simulink model "VR_acquisition_serial"  (Simulink 8.4)
settings: Solver=ode45  StartTime=0.0  StopTime=inf  RelTol=1e-3
libraries: vrlib x8, aerolibtransform2 x4, aerolibconvert2 x3
settings Model: Creator=AMANALLAH  LastModifiedBy=AMANALLAH
settings DataIOCC: SignalLoggingSaveFormat=Dataset
settings OptimizationCC: ExpressionDepthLimit=128
settings DebuggingCC: UnderspecifiedInitializationDetection=Simplified  MergeDetectMultiDrivingBlocksExec=error  FcnCallInpInsideContextMsg=EnableAllAsError  StateNameClashWarn=none
settings GRTTargetCC: CombineOutputUpdateFcns=on  GRTInterface=off

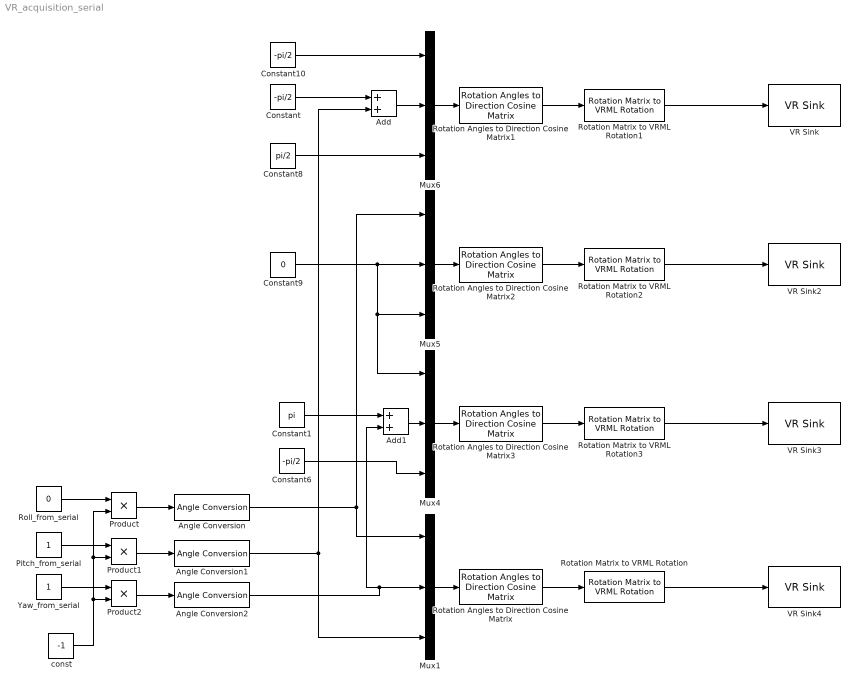
== system VR_acquisition_serial ==
  Add : Sum
  Add1 : Sum
  Angle Conversion : aerolibconvert2/Angle Conversion  IU=deg  OU=rad
  Angle Conversion1 : aerolibconvert2/Angle Conversion  IU=deg  OU=rad
  Angle Conversion2 : aerolibconvert2/Angle Conversion  IU=deg  OU=rad
  Constant : Constant  Value=-pi/2
  Constant1 : Constant  Value=pi
  Constant10 : Constant  Value=-pi/2
  Constant6 : Constant  Value=-pi/2
  Constant8 : Constant  Value=pi/2
  Constant9 : Constant  Value=0
  Mux{1,4..6} (4 alike) : Mux  Inputs=3
  Pitch_from_serial : Constant
  Product : Product
  Product1 : Product
  Product2 : Product
  Roll_from_serial : Constant  Value=0
  Rotation Angles to Direction Cosine Matrix{,1..3} (4 alike) : aerolibtransform2/Rotation Angles to Direction Cosine Matrix  rotationOrder=ZYX
  Rotation Matrix to VRML Rotation{,1..3} (4 alike) : vrlib/Utilities/Rotation Matrix to VRML Rotation  maxzero=1e-12
  VR Sink : vrlib/VR Sink  InstantiateOnLoad=on  SampleTime=0.1  ViewEnable=on  RemoteChange=off  RemoteView=off  FieldsWritten=Airplane.rotation.4.1.1.double  WorldFileName=spitfire_3d_pitch.WRL  AutoView=off  VideoDimensions=[]  AllowVariableSize=off
  VR Sink2 : vrlib/VR Sink  InstantiateOnLoad=on  SampleTime=0.1  ViewEnable=on  RemoteChange=off  RemoteView=off  FieldsWritten=Airplane.rotation.4.1.1.double  WorldFileName=spitfire_3d_roll.WRL  AutoView=off  VideoDimensions=[]  AllowVariableSize=off
  VR Sink3 : vrlib/VR Sink  InstantiateOnLoad=on  SampleTime=0.1  ViewEnable=on  RemoteChange=off  RemoteView=off  FieldsWritten=Airplane.rotation.4.1.1.double  WorldFileName=spitfire_3d_yaw.WRL  AutoView=off  VideoDimensions=[]  AllowVariableSize=off
  VR Sink4 : vrlib/VR Sink  InstantiateOnLoad=on  SampleTime=0.1  ViewEnable=on  RemoteChange=off  RemoteView=off  FieldsWritten=Airplane.rotation.4.1.1.double  WorldFileName=spitfire_3d.WRL  AutoView=off  VideoDimensions=[]  AllowVariableSize=off  FigureProperties="{'Position', 'Name', 'Viewpoint', 'CameraBound', 'CameraDirection', 'CameraPosition', 'CameraUpVector', 'ZoomFactor', 'Antialiasing', 'Headlight', 'Lighting', 'NavPanel', 'Sound', 'StatusBar', 'Stereo3D', 'Stereo3DCameraOffset', 'Stereo3DHIT', 'ToolBar', 'Textures', 'Transparency', 'Triad', 'Wireframe', 'NavZones', 'NavMode', 'NavSpeed', 'CaptureFileFormat', 'CaptureFileName', 'Record2DCompressMethod', 'Record2DCompressQuality', 'Record2D', 'Record2DFileName', 'Record2DFPS'; [4.9900000000000000e+02   1.5700000000000000e+02   5.7600000000000000e+02   3.8000000000000000e+02], '', '_untitled_1', 'on', [0.0000000000000000e+00   0.0000000000000000e+00  -1.0000000000000000e+00], [0.0000000000000000e+00   0.0000000000000000e+00   0.0000000000000000e+00], [0.0000000000000000e+00   1.0000000000000000e+00   0.0000000000000000e+00], [1.0000000000000000e+00], 'on', 'on', 'on', 'halfbar', 'on', 'on', 'off', [1.0000000149011612e-01], [0.0000000000000000e+00], 'on', 'on', 'on', 'none', 'off', 'off', 'fly', 'normal', 'tif', '%f_anim_%n.tif', 'auto', [7.5000000000000000e+01], 'off', '%f_anim_%n.avi', 'auto'}"
  Yaw_from_serial : Constant
  const : Constant  Value=-1
  wires:
  Rotation Matrix to VRML Rotation/1 -> VR Sink4/1
  Rotation Angles to Direction Cosine Matrix/1 -> Rotation Matrix to VRML Rotation/1
  Mux1/1 -> Rotation Angles to Direction Cosine Matrix/1
  Mux6/1 -> Rotation Angles to Direction Cosine Matrix1/1
  Rotation Angles to Direction Cosine Matrix1/1 -> Rotation Matrix to VRML Rotation1/1
  Rotation Matrix to VRML Rotation1/1 -> VR Sink/1
  Mux5/1 -> Rotation Angles to Direction Cosine Matrix2/1
  Rotation Angles to Direction Cosine Matrix2/1 -> Rotation Matrix to VRML Rotation2/1
  Rotation Matrix to VRML Rotation2/1 -> VR Sink2/1
  Mux4/1 -> Rotation Angles to Direction Cosine Matrix3/1
  Rotation Angles to Direction Cosine Matrix3/1 -> Rotation Matrix to VRML Rotation3/1
  Rotation Matrix to VRML Rotation3/1 -> VR Sink3/1
  Constant9/1 -> Mux4/1, Mux5/3, Mux5/2
  Constant6/1 -> Mux4/3
  Constant10/1 -> Mux6/1
  Constant8/1 -> Mux6/3
  Constant/1 -> Add/1
  Add/1 -> Mux6/2
  Add1/1 -> Mux4/2
  Constant1/1 -> Add1/1
  Angle Conversion/1 -> Mux1/1, Mux5/1
  Angle Conversion2/1 -> Add1/2, Mux1/2
  Angle Conversion1/1 -> Add/2, Mux1/3
  Roll_from_serial/1 -> Product/1
  Product/1 -> Angle Conversion/1
  Product1/1 -> Angle Conversion1/1
  Product2/1 -> Angle Conversion2/1
  Pitch_from_serial/1 -> Product1/1
  Yaw_from_serial/1 -> Product2/1
  const/1 -> Product/2, Product1/2, Product2/2
